simulink model "SF034A_AssiPahFwl"  (R2013b)
settings: Solver=FixedStepDiscrete  SolverMode=SingleTasking  StartTime=0.0  StopTime=1  FixedStep=0.002  RelTol=1e-3
values from neighbouring files (symbols this model uses):
  ARCHGLBPRM_2MILLISEC_SEC_F32 = DataDict.Constant    [SF034A_AssiPahFwl_DataDict.m]
  AssiPahFwlDiRcvr = DataDict.Calibration    [SF034A_AssiPahFwl_DataDict.m]
  AssiPahFwlHysCmpLim = DataDict.Calibration    [SF034A_AssiPahFwl_DataDict.m]
  AssiPahFwlRestoreThd = DataDict.Calibration    [SF034A_AssiPahFwl_DataDict.m]
  BasAssiPahFwlOverLimDiagcFailStep = DataDict.Calibration    [SF034A_AssiPahFwl_DataDict.m]
  BasAssiPahFwlOverLimDiagcPassStep = DataDict.Calibration    [SF034A_AssiPahFwl_DataDict.m]
  BASASSIREACHED_CNT_U08 = DataDict.Constant    [SF034A_AssiPahFwl_DataDict.m]
  HiFrqAssiPahFwlOverLimDiagcFailStep = DataDict.Calibration    [SF034A_AssiPahFwl_DataDict.m]
  HiFrqAssiPahFwlOverLimDiagcPassStep = DataDict.Calibration    [SF034A_AssiPahFwl_DataDict.m]
  HIFRQASSIREACHED_CNT_U08 = DataDict.Constant    [SF034A_AssiPahFwl_DataDict.m]
undefined symbols (not defined in the file or in its folder): MfgEnaSt1, NtcNr1, NtcSts1, sigbuilder_block, SigQlfr1
libraries: simulink x23, Fil x8, NxtrLim x5, FixdToFloat x5, BilnrIntrpnMplX x4, FloatToFixd x4, NxtrAbslt x2, LnrIntrpn x1, NxtrSign x1
(part 3 of 3)

== system SF034A_AssiPahFwl/AssiPahFwl/AssiPahFwlPer1/Normal_Firewall_Operation/Set_Faults/Set AssiFwlFlt/AssiFwlFltMode/CopyRight2 ==

== system SF034A_AssiPahFwl/AssiPahFwl/AssiPahFwlPer1/Normal_Firewall_Operation/Set_Faults/Set AssiFwlFlt/AssiFwlFltMode/SetNtcSts ==
  note: Note:
      |
      | - "ISO Fault Debounce Design" Simulink block intent to use here for Simulation purpose only. Do not Code this block
  NtcNr : Inport
  NtcStInfo : Inport  Port=2
  NtcSts : Inport  Port=3
  DebStep : Inport  Port=4
  CopyRight2 : Subsystem  Description=|  mask(Copyright Information){none=on}
      | Copyright info block.                                               
      |                                                                     
      | Place copyright information at the top of every subsystem in design.
      mask prompts: none "No parameters"
      mask help: Place copyright information at the top of every subsystem in design.
      mask Display:
      | NxtrConf = 'Nexteer Confidential';
      | 
      | sys = bdroot; %handle for the current model ("system")
      | first = get_param(sys,'Created');
      | if(isempty(first))
      |     first = datestr(now,'yyyy');
      | else
      |     first = first(end-3:end);  %year is last four digits
      | end
      | 
      | last = get_param(sys,'LastModifiedDate');
      | if isempty(last)
      |     last = datestr(now,'yyyy');
      | else
      |     last = last(end-3:end);
      | end
      | 
      | if strcmp(first,last)
      |     fprintf('%s -- Copyright %s Nexteer',NxtrConf,first)
      | else
      |     fprintf('%s -- %s%s- %s Nexteer',NxtrConf,char(169),first,last)
      | end
  Data Store Write : DataStoreWrite  DataStoreName=Ntc0x0C9Qlfr
  Data Type Conversion : DataTypeConversion  OutDataTypeStr=Enum: SigQlfr1
  Ground : Ground
  ISO Fault Debounce Design : Stateflow chart  TreatAsAtomicUnit=on
      settings: AttributesFormatString=|
      | Simulation Purpose Only.
      | Do Not Code this block
      | Diagnostic Manager Owns this requirement
  Terminator : Terminator
  Terminator1 : Terminator
  wires:
  Ground/1 -> ISO Fault Debounce Design/3(SvcClr)
  ISO Fault Debounce Design/1(Qualifier) -> Data Type Conversion/1
  DebStep/1 -> ISO Fault Debounce Design/2(DebStep)
  NtcNr/1 -> Terminator/1
  NtcStInfo/1 -> Terminator1/1
  NtcSts/1 -> ISO Fault Debounce Design/1(NtcSts)
  Data Type Conversion/1 -> Data Store Write/1

== system SF034A_AssiPahFwl/AssiPahFwl/AssiPahFwlPer1/Normal_Firewall_Operation/Set_Faults/Set AssiFwlFlt/If Action Subsystem/CopyRight2 ==

== system SF034A_AssiPahFwl/AssiPahFwl/AssiPahFwlPer1/Normal_Firewall_Operation/Set_Faults/Set AssiFwlFlt/If Action Subsystem1/CopyRight2 ==

== system SF034A_AssiPahFwl/AssiPahFwl/AssiPahFwlPer1/Normal_Firewall_Operation/Set_Faults/Set AssiFwlFlt/If Action Subsystem2/CopyRight2 ==

== system SF034A_AssiPahFwl/AssiPahFwl/AssiPahFwlPer1/Normal_Firewall_Operation/Set_Faults/Set AssiFwlFlt/If Action Subsystem3/CopyRight2 ==

== system SF034A_AssiPahFwl/AssiPahFwl/AssiPahFwlPer1/Normal_Firewall_Operation/Set_Faults/Set AssiFwlFlt/AssiFwlFltMode/SetNtcSts/CopyRight2 ==

== stateflow chart SF034A_AssiPahFwl/AssiPahFwl/AssiPahFwlPer1/Normal_Firewall_Operation/Debounce_HiFreqAsst_Overboundary/SetNtcSts/SetNtcSts/ISO Fault Debounce Design ==
  note: NTCSTS_PASSD           (0)
      | NTCSTS_FAILD             (1)
      | NTCSTS_PREPASSD   (2)
      | NTCSTS_PREFAILD     (3)
      |
      | SIGQLFR_NORES        (0)
      | SIGQLFR_PASSD         (1)
      | SIGQLFR_FAILD           (2)
  note: Pass Loop
  note: Fail Loop
  note: 
  (default) -> (junction 89)
  (junction 89) -> (junction 95) [order 1] : [NtcSts ==3]
  (junction 89) -> (junction 93) [order 2] : [NtcSts ==2]
  (junction 89) -> (junction 141) [order 3] : [NtcSts ==1]
      | { ErrAcc = 32767;
      | Qualifier =2;
      |  }
  (junction 89) -> (junction 141) [order 4] : [NtcSts ==0]
      | { ErrAcc = -32768;
      | Qualifier=1;
      | }
  (junction 95) -> (junction 103) [order 2]
  (junction 95) -> (junction 111) [order 1] : [ErrAcc <=0]
      | {ErrAcc = DebStep;}
  (junction 93) -> (junction 123) [order 2] : {
      | ErrAcc = ErrAcc - DebStep;
      | }
  (junction 93) -> (junction 123) [order 1] : [(ErrAcc - DebStep) <= -32768]
      | { ErrAcc = -32768;
      | Qualifier=1;
      | }
  (junction 103) -> (junction 111) [order 1] : [(ErrAcc + DebStep) <32767]
      | {ErrAcc = ErrAcc + DebStep;}
  (junction 103) -> (junction 111) [order 2] : {ErrAcc = 32767;
      | Qualifier =2;}
  (junction 123) -> (junction 141)
  (junction 111) -> (junction 141)
  (junction 141) -> (junction 159) [order 2] : {ErrAcc = 0;
      | Qualifier =0;
      | }
  (junction 141) -> (junction 159) [order 1] : [SvcClr ==0]
  data: NtcSts input Enum: NtcSts1; Qualifier output uint8; DebStep input uint16; ErrAcc local single; SvcClr input

== stateflow chart SF034A_AssiPahFwl/AssiPahFwl/AssiPahFwlPer1/Normal_Firewall_Operation/Debounce_HiFreqAsst_Overboundary/SetNtcSts1/SetNtcSts/ISO Fault Debounce Design ==
  note: NTCSTS_PASSD           (0)
      | NTCSTS_FAILD             (1)
      | NTCSTS_PREPASSD   (2)
      | NTCSTS_PREFAILD     (3)
      |
      | SIGQLFR_NORES        (0)
      | SIGQLFR_PASSD         (1)
      | SIGQLFR_FAILD           (2)
  note: Pass Loop
  note: Fail Loop
  note: 
  (default) -> (junction 89)
  (junction 89) -> (junction 95) [order 1] : [NtcSts ==3]
  (junction 89) -> (junction 93) [order 2] : [NtcSts ==2]
  (junction 89) -> (junction 141) [order 3] : [NtcSts ==1]
      | { ErrAcc = 32767;
      | Qualifier =2;
      |  }
  (junction 89) -> (junction 141) [order 4] : [NtcSts ==0]
      | { ErrAcc = -32768;
      | Qualifier=1;
      | }
  (junction 95) -> (junction 103) [order 2]
  (junction 95) -> (junction 111) [order 1] : [ErrAcc <=0]
      | {ErrAcc = DebStep;}
  (junction 93) -> (junction 123) [order 2] : {
      | ErrAcc = ErrAcc - DebStep;
      | }
  (junction 93) -> (junction 123) [order 1] : [(ErrAcc - DebStep) <= -32768]
      | { ErrAcc = -32768;
      | Qualifier=1;
      | }
  (junction 103) -> (junction 111) [order 1] : [(ErrAcc + DebStep) <32767]
      | {ErrAcc = ErrAcc + DebStep;}
  (junction 103) -> (junction 111) [order 2] : {ErrAcc = 32767;
      | Qualifier =2;}
  (junction 123) -> (junction 141)
  (junction 111) -> (junction 141)
  (junction 141) -> (junction 159) [order 2] : {ErrAcc = 0;
      | Qualifier =0;
      | }
  (junction 141) -> (junction 159) [order 1] : [SvcClr ==0]
  data: NtcSts input Enum: NtcSts1; Qualifier output uint8; DebStep input uint16; ErrAcc local single; SvcClr input

== stateflow chart SF034A_AssiPahFwl/AssiPahFwl/AssiPahFwlPer1/Normal_Firewall_Operation/Debounce_BaseAssist_Overboundary/SetNtcSts/SetNtcSts/ISO Fault Debounce Design ==
  note: NTCSTS_PASSD           (0)
      | NTCSTS_FAILD             (1)
      | NTCSTS_PREPASSD   (2)
      | NTCSTS_PREFAILD     (3)
      |
      | SIGQLFR_NORES        (0)
      | SIGQLFR_PASSD         (1)
      | SIGQLFR_FAILD           (2)
  note: Pass Loop
  note: Fail Loop
  note: 
  (default) -> (junction 89)
  (junction 89) -> (junction 95) [order 1] : [NtcSts ==3]
  (junction 89) -> (junction 93) [order 2] : [NtcSts ==2]
  (junction 89) -> (junction 141) [order 3] : [NtcSts ==1]
      | { ErrAcc = 32767;
      | Qualifier =2;
      |  }
  (junction 89) -> (junction 141) [order 4] : [NtcSts ==0]
      | { ErrAcc = -32768;
      | Qualifier=1;
      | }
  (junction 95) -> (junction 103) [order 2]
  (junction 95) -> (junction 111) [order 1] : [ErrAcc <=0]
      | {ErrAcc = DebStep;}
  (junction 93) -> (junction 123) [order 2] : {
      | ErrAcc = ErrAcc - DebStep;
      | }
  (junction 93) -> (junction 123) [order 1] : [(ErrAcc - DebStep) <= -32768]
      | { ErrAcc = -32768;
      | Qualifier=1;
      | }
  (junction 103) -> (junction 111) [order 1] : [(ErrAcc + DebStep) <32767]
      | {ErrAcc = ErrAcc + DebStep;}
  (junction 103) -> (junction 111) [order 2] : {ErrAcc = 32767;
      | Qualifier =2;}
  (junction 123) -> (junction 141)
  (junction 111) -> (junction 141)
  (junction 141) -> (junction 159) [order 2] : {ErrAcc = 0;
      | Qualifier =0;
      | }
  (junction 141) -> (junction 159) [order 1] : [SvcClr ==0]
  data: NtcSts input Enum: NtcSts1; Qualifier output uint8; DebStep input uint16; ErrAcc local single; SvcClr input

== stateflow chart SF034A_AssiPahFwl/AssiPahFwl/AssiPahFwlPer1/Normal_Firewall_Operation/Debounce_BaseAssist_Overboundary/SetNtcSts1/SetNtcSts/ISO Fault Debounce Design ==
  note: NTCSTS_PASSD           (0)
      | NTCSTS_FAILD             (1)
      | NTCSTS_PREPASSD   (2)
      | NTCSTS_PREFAILD     (3)
      |
      | SIGQLFR_NORES        (0)
      | SIGQLFR_PASSD         (1)
      | SIGQLFR_FAILD           (2)
  note: Pass Loop
  note: Fail Loop
  note: 
  (default) -> (junction 89)
  (junction 89) -> (junction 95) [order 1] : [NtcSts ==3]
  (junction 89) -> (junction 93) [order 2] : [NtcSts ==2]
  (junction 89) -> (junction 141) [order 3] : [NtcSts ==1]
      | { ErrAcc = 32767;
      | Qualifier =2;
      |  }
  (junction 89) -> (junction 141) [order 4] : [NtcSts ==0]
      | { ErrAcc = -32768;
      | Qualifier=1;
      | }
  (junction 95) -> (junction 103) [order 2]
  (junction 95) -> (junction 111) [order 1] : [ErrAcc <=0]
      | {ErrAcc = DebStep;}
  (junction 93) -> (junction 123) [order 2] : {
      | ErrAcc = ErrAcc - DebStep;
      | }
  (junction 93) -> (junction 123) [order 1] : [(ErrAcc - DebStep) <= -32768]
      | { ErrAcc = -32768;
      | Qualifier=1;
      | }
  (junction 103) -> (junction 111) [order 1] : [(ErrAcc + DebStep) <32767]
      | {ErrAcc = ErrAcc + DebStep;}
  (junction 103) -> (junction 111) [order 2] : {ErrAcc = 32767;
      | Qualifier =2;}
  (junction 123) -> (junction 141)
  (junction 111) -> (junction 141)
  (junction 141) -> (junction 159) [order 2] : {ErrAcc = 0;
      | Qualifier =0;
      | }
  (junction 141) -> (junction 159) [order 1] : [SvcClr ==0]
  data: NtcSts input Enum: NtcSts1; Qualifier output uint8; DebStep input uint16; ErrAcc local single; SvcClr input

== stateflow chart SF034A_AssiPahFwl/AssiPahFwl/AssiPahFwlPer1/Normal_Firewall_Operation/Set_Faults/Set AssiFwlFlt/AssiFwlFltMode/SetNtcSts/ISO Fault Debounce Design ==
  note: NTCSTS_PASSD           (0)
      | NTCSTS_FAILD             (1)
      | NTCSTS_PREPASSD   (2)
      | NTCSTS_PREFAILD     (3)
      |
      | SIGQLFR_NORES        (0)
      | SIGQLFR_PASSD         (1)
      | SIGQLFR_FAILD           (2)
  note: Pass Loop
  note: Fail Loop
  note: 
  (default) -> (junction 89)
  (junction 89) -> (junction 95) [order 1] : [NtcSts ==3]
  (junction 89) -> (junction 93) [order 2] : [NtcSts ==2]
  (junction 89) -> (junction 141) [order 3] : [NtcSts ==1]
      | { ErrAcc = 32767;
      | Qualifier =2;
      |  }
  (junction 89) -> (junction 141) [order 4] : [NtcSts ==0]
      | { ErrAcc = -32768;
      | Qualifier=1;
      | }
  (junction 95) -> (junction 103) [order 2]
  (junction 95) -> (junction 111) [order 1] : [ErrAcc <=0]
      | {ErrAcc = DebStep;}
  (junction 93) -> (junction 123) [order 2] : {
      | ErrAcc = ErrAcc - DebStep;
      | }
  (junction 93) -> (junction 123) [order 1] : [(ErrAcc - DebStep) <= -32768]
      | { ErrAcc = -32768;
      | Qualifier=1;
      | }
  (junction 103) -> (junction 111) [order 1] : [(ErrAcc + DebStep) <32767]
      | {ErrAcc = ErrAcc + DebStep;}
  (junction 103) -> (junction 111) [order 2] : {ErrAcc = 32767;
      | Qualifier =2;}
  (junction 123) -> (junction 141)
  (junction 111) -> (junction 141)
  (junction 141) -> (junction 159) [order 2] : {ErrAcc = 0;
      | Qualifier =0;
      | }
  (junction 141) -> (junction 159) [order 1] : [SvcClr ==0]
  data: NtcSts input Enum: NtcSts1; Qualifier output uint8; DebStep input uint16; ErrAcc local single; SvcClr input

== stateflow chart SF034A_AssiPahFwl/AssiPahFwl/AssiPahFwlInit1/AssiFwlFltMode/SetNtcSts/ISO Fault Debounce Design ==
  note: NTCSTS_PASSD           (0)
      | NTCSTS_FAILD             (1)
      | NTCSTS_PREPASSD   (2)
      | NTCSTS_PREFAILD     (3)
      |
      | SIGQLFR_NORES        (0)
      | SIGQLFR_PASSD         (1)
      | SIGQLFR_FAILD           (2)
  note: Pass Loop
  note: Fail Loop
  note: 
  (default) -> (junction 89)
  (junction 89) -> (junction 95) [order 1] : [NtcSts ==3]
  (junction 89) -> (junction 93) [order 2] : [NtcSts ==2]
  (junction 89) -> (junction 141) [order 3] : [NtcSts ==1]
      | { ErrAcc = 32767;
      | Qualifier =2;
      |  }
  (junction 89) -> (junction 141) [order 4] : [NtcSts ==0]
      | { ErrAcc = -32768;
      | Qualifier=1;
      | }
  (junction 95) -> (junction 103) [order 2]
  (junction 95) -> (junction 111) [order 1] : [ErrAcc <=0]
      | {ErrAcc = DebStep;}
  (junction 93) -> (junction 123) [order 2] : {
      | ErrAcc = ErrAcc - DebStep;
      | }
  (junction 93) -> (junction 123) [order 1] : [(ErrAcc - DebStep) <= -32768]
      | { ErrAcc = -32768;
      | Qualifier=1;
      | }
  (junction 103) -> (junction 111) [order 1] : [(ErrAcc + DebStep) <32767]
      | {ErrAcc = ErrAcc + DebStep;}
  (junction 103) -> (junction 111) [order 2] : {ErrAcc = 32767;
      | Qualifier =2;}
  (junction 123) -> (junction 141)
  (junction 111) -> (junction 141)
  (junction 141) -> (junction 159) [order 2] : {ErrAcc = 0;
      | Qualifier =0;
      | }
  (junction 141) -> (junction 159) [order 1] : [SvcClr ==0]
  data: NtcSts input Enum: NtcSts1; Qualifier output uint8; DebStep input uint16; ErrAcc local single; SvcClr input

== stateflow chart SF034A_AssiPahFwl/AssiPahFwl/AssiPahFwlInit1/BaseAssistFwlReached/SetNtcSts/ISO Fault Debounce Design ==
  note: NTCSTS_PASSD           (0)
      | NTCSTS_FAILD             (1)
      | NTCSTS_PREPASSD   (2)
      | NTCSTS_PREFAILD     (3)
      |
      | SIGQLFR_NORES        (0)
      | SIGQLFR_PASSD         (1)
      | SIGQLFR_FAILD           (2)
  note: Pass Loop
  note: Fail Loop
  note: 
  (default) -> (junction 89)
  (junction 89) -> (junction 95) [order 1] : [NtcSts ==3]
  (junction 89) -> (junction 93) [order 2] : [NtcSts ==2]
  (junction 89) -> (junction 141) [order 3] : [NtcSts ==1]
      | { ErrAcc = 32767;
      | Qualifier =2;
      |  }
  (junction 89) -> (junction 141) [order 4] : [NtcSts ==0]
      | { ErrAcc = -32768;
      | Qualifier=1;
      | }
  (junction 95) -> (junction 103) [order 2]
  (junction 95) -> (junction 111) [order 1] : [ErrAcc <=0]
      | {ErrAcc = DebStep;}
  (junction 93) -> (junction 123) [order 2] : {
      | ErrAcc = ErrAcc - DebStep;
      | }
  (junction 93) -> (junction 123) [order 1] : [(ErrAcc - DebStep) <= -32768]
      | { ErrAcc = -32768;
      | Qualifier=1;
      | }
  (junction 103) -> (junction 111) [order 1] : [(ErrAcc + DebStep) <32767]
      | {ErrAcc = ErrAcc + DebStep;}
  (junction 103) -> (junction 111) [order 2] : {ErrAcc = 32767;
      | Qualifier =2;}
  (junction 123) -> (junction 141)
  (junction 111) -> (junction 141)
  (junction 141) -> (junction 159) [order 2] : {ErrAcc = 0;
      | Qualifier =0;
      | }
  (junction 141) -> (junction 159) [order 1] : [SvcClr ==0]
  data: NtcSts input Enum: NtcSts1; Qualifier output uint8; DebStep input uint16; ErrAcc local single; SvcClr input

== stateflow chart SF034A_AssiPahFwl/AssiPahFwl/AssiPahFwlInit1/HiFrqAssiFwlReached/SetNtcSts/ISO Fault Debounce Design ==
  note: NTCSTS_PASSD           (0)
      | NTCSTS_FAILD             (1)
      | NTCSTS_PREPASSD   (2)
      | NTCSTS_PREFAILD     (3)
      |
      | SIGQLFR_NORES        (0)
      | SIGQLFR_PASSD         (1)
      | SIGQLFR_FAILD           (2)
  note: Pass Loop
  note: Fail Loop
  note: 
  (default) -> (junction 89)
  (junction 89) -> (junction 95) [order 1] : [NtcSts ==3]
  (junction 89) -> (junction 93) [order 2] : [NtcSts ==2]
  (junction 89) -> (junction 141) [order 3] : [NtcSts ==1]
      | { ErrAcc = 32767;
      | Qualifier =2;
      |  }
  (junction 89) -> (junction 141) [order 4] : [NtcSts ==0]
      | { ErrAcc = -32768;
      | Qualifier=1;
      | }
  (junction 95) -> (junction 103) [order 2]
  (junction 95) -> (junction 111) [order 1] : [ErrAcc <=0]
      | {ErrAcc = DebStep;}
  (junction 93) -> (junction 123) [order 2] : {
      | ErrAcc = ErrAcc - DebStep;
      | }
  (junction 93) -> (junction 123) [order 1] : [(ErrAcc - DebStep) <= -32768]
      | { ErrAcc = -32768;
      | Qualifier=1;
      | }
  (junction 103) -> (junction 111) [order 1] : [(ErrAcc + DebStep) <32767]
      | {ErrAcc = ErrAcc + DebStep;}
  (junction 103) -> (junction 111) [order 2] : {ErrAcc = 32767;
      | Qualifier =2;}
  (junction 123) -> (junction 141)
  (junction 111) -> (junction 141)
  (junction 141) -> (junction 159) [order 2] : {ErrAcc = 0;
      | Qualifier =0;
      | }
  (junction 141) -> (junction 159) [order 1] : [SvcClr ==0]
  data: NtcSts input Enum: NtcSts1; Qualifier output uint8; DebStep input uint16; ErrAcc local single; SvcClr input
